simulink library "myLibrary"  (R2023b)
settings: Solver=VariableStepAuto  StartTime=0.0  StopTime=10.0  RelTol=1e-3
undefined symbols (not defined in the file): Cac_n1, ctrl1, Da, Discrete, dtha, ee_sli_rtmsupport, FA, gcbh, Ha, Ini, init_DCline, init_IPC, init_line, init_load, init_SG, init_shunt, init_TH, init_trafo, init_VSC, initMachineBlocks, Ka, Lf, Llkd_pu, Llkq1_pu, magnitude, NET, P, plots_step, q0, Rac_n1, Radd, Rkd_pu, Rkq1_pu, Rload_add, sim_config, sps_rtmsupport, spsSteamTurbineModel, T_DC_NET, T_global, T_IPC, T_load, T_NET, T_SG, T_shunt, T_STATCOM, T_TH, T_trafo, T_VSC, Ts, tstep, Udiff_a, V1
libraries: spsSeriesRLCBranchLib x105, eeGeneralControl x72, $bdroot x70, spsCurrentMeasurementLib x48, spsParallelRLCBranchLib x39, spsVoltageMeasurementLib x33, spsControlledVoltageSourceLib x27, spsFirstOrderFilterLib x16, dspsigops x6, spsThreePhaseVIMeasurementLib x5, spsPLL3phLib x4, spsThreePhaseBreakerLib x3
(part 12 of 12)

== system myLibrary/SG_step/Governor-Turbine/Steam Turbine and Governor/Model/4 mass shaft/3 masses/Mass4/Prediction ==
  I : Inport
  Gain1 : Gain  Gain=2  SaturateOnIntegerOverflow=on  OutDataTypeStr=Inherit: Same as input  ParamDataTypeStr=Inherit: Same as input
  Sum1 : Sum  Inputs=+-  InputSameDT=on  SaturateOnIntegerOverflow=on  OutDataTypeStr=Inherit: Same as first input
  Unit Delay3 : UnitDelay  InitialCondition=dth0  SampleTime=Ts  HasFrameUpgradeWarning=on
  O : Outport
  wires:
  Sum1/1 -> O/1
  Unit Delay3/1 -> Sum1/2
  Gain1/1 -> Sum1/1
  I/1 -> Unit Delay3/1, Gain1/1

== system myLibrary/SG_step/Governor-Turbine/Steam Turbine and Governor/Model/4 mass shaft/4 masses/Mass2/Prediction ==
  I : Inport
  Gain1 : Gain  Gain=2  SaturateOnIntegerOverflow=on  OutDataTypeStr=Inherit: Same as input  ParamDataTypeStr=Inherit: Same as input
  Sum1 : Sum  Inputs=+-  InputSameDT=on  SaturateOnIntegerOverflow=on  OutDataTypeStr=Inherit: Same as first input
  Unit Delay3 : UnitDelay  InitialCondition=initSG.delta2  SampleTime=Ts  HasFrameUpgradeWarning=on
  O : Outport
  wires:
  I/1 -> Gain1/1, Unit Delay3/1
  Gain1/1 -> Sum1/1
  Unit Delay3/1 -> Sum1/2
  Sum1/1 -> O/1

== system myLibrary/SG_step/Governor-Turbine/Steam Turbine and Governor/Model/4 mass shaft/4 masses/Mass3/Prediction ==
  I : Inport
  Gain1 : Gain  Gain=2  SaturateOnIntegerOverflow=on  OutDataTypeStr=Inherit: Same as input  ParamDataTypeStr=Inherit: Same as input
  Sum1 : Sum  Inputs=+-  InputSameDT=on  SaturateOnIntegerOverflow=on  OutDataTypeStr=Inherit: Same as first input
  Unit Delay3 : UnitDelay  InitialCondition=initSG.delta3  SampleTime=Ts  HasFrameUpgradeWarning=on
  O : Outport
  wires:
  Sum1/1 -> O/1
  Unit Delay3/1 -> Sum1/2
  Gain1/1 -> Sum1/1
  I/1 -> Unit Delay3/1, Gain1/1

== system myLibrary/SG_step/Governor-Turbine/Steam Turbine and Governor/Model/4 mass shaft/4 masses/Mass4/Prediction ==
  I : Inport
  Gain1 : Gain  Gain=2  SaturateOnIntegerOverflow=on  OutDataTypeStr=Inherit: Same as input  ParamDataTypeStr=Inherit: Same as input
  Sum1 : Sum  Inputs=+-  InputSameDT=on  SaturateOnIntegerOverflow=on  OutDataTypeStr=Inherit: Same as first input
  Unit Delay3 : UnitDelay  InitialCondition=initSG.delta4  SampleTime=Ts  HasFrameUpgradeWarning=on
  O : Outport
  wires:
  I/1 -> Gain1/1, Unit Delay3/1
  Gain1/1 -> Sum1/1
  Unit Delay3/1 -> Sum1/2
  Sum1/1 -> O/1

== system myLibrary/SG_step/Governor-Turbine/Steam Turbine and Governor/Model/4 mass shaft/4 masses/Mass5/Prediction ==
  I : Inport
  Gain1 : Gain  Gain=2  SaturateOnIntegerOverflow=on  OutDataTypeStr=Inherit: Same as input  ParamDataTypeStr=Inherit: Same as input
  Sum1 : Sum  Inputs=+-  InputSameDT=on  SaturateOnIntegerOverflow=on  OutDataTypeStr=Inherit: Same as first input
  Unit Delay3 : UnitDelay  InitialCondition=initSG.delta5  SampleTime=Ts  HasFrameUpgradeWarning=on
  O : Outport
  wires:
  Sum1/1 -> O/1
  Unit Delay3/1 -> Sum1/2
  Gain1/1 -> Sum1/1
  I/1 -> Unit Delay3/1, Gain1/1

== matlab function myLibrary/SG/Exciter/Exciter ST4B/Fex/fex ==
  data: I_N input; F_EX output
function F_EX = fex(I_N)
% AVRFEX Rectifier regulation characteristic based on: IEEE Recommended
% Practice for Excitation System Models for Power System Stability Studies,
% IEEE Std 421.5-2006,Annex D, Rectifier Regulation

F_EX = ee.control.sm.fex(I_N);

end

== matlab function myLibrary/SG_step/Exciter/Exciter ST4B/Fex/fex ==
  data: I_N input; F_EX output
function F_EX = fex(I_N)
% AVRFEX Rectifier regulation characteristic based on: IEEE Recommended
% Practice for Excitation System Models for Power System Stability Studies,
% IEEE Std 421.5-2006,Annex D, Rectifier Regulation

F_EX = ee.control.sm.fex(I_N);

end
